simulink model "sixdof"  (R2019a)
settings: Solver=VariableStepAuto  StartTime=0.0  StopTime=15  RelTol=1e-3
InitFcn:
  | HeightAboveSeaLevel = 400 * rand;
  | Temperature = 288.15 + 30 * (rand - 0.5);
  | Pressure = 	101325 + 6000 * (rand - 0.5);
  | 
  | GustStart = 5 * rand;
  | GustLength = [100 + 50 * (rand - 0.5), 100 + 50 * (rand - 0.5), 100 + 50 * (rand - 0.5)];
  | GuestAmplitude = [ 10 * (rand - 0.5), 10 * (rand - 0.5),  10 * (rand - 0.5)];
  | 
  | ShearSpeed = 20 * rand;
  | ShearDirection = 360 * rand;
  | 
  | HeightAboveSeaLevel = 5.4419142084;
  | Temperature = 288.15;
  | Pressure = 	101325;
  | 
  | GustStart = 2.5;
  | GustLength = [100, 100, 100];
  | GuestAmplitude = [ 2.5, -2.5,  1];
  | 
  | ShearSpeed = 10;
  | ShearDirection = 180;
values from neighbouring files (symbols this model uses):
  cg = temp(4)    [NonlinearStateEstimationForActuatorDelay.m]
  D = zeros(size(B))    [RocketOutputFunction.m]    (also in StateSpaceController.m = zeros(13, 3); TimeDelayCompensationElevator.m = [0; 0])
  F = eye(6)    [MEKFAttitudeOnly.m]
  I = reshape(x(1:9), [3 3])    [AdaptiveLQR.m]    (also in MEKF.m = diag([0.08 0.08 0.002]); MEKFAttitudeOnly.m = diag([0.08 0.08 0.002]); MEKF_old.m = diag([0.08 0.08 0.002]); NonlinearStateEstimationForActuatorDelay.m = diag([Ixx, Ixx, Izz]))
  Ki2 = lqr(Ai2, Bi2, Q, R)    [StateSpaceController.m]
  mass = 1.0565    [ImpactVelocityNotParallelMatlab.m]    (also in NonlinearStateEstimationForActuatorDelay.m = temp(1); OneDLanding.m; RunImpactVelocityParforCompiled.m; Tracker.m = 1.0616753546)
  q = x(13:16)    [AdaptiveLQR.m]    (also in MEKF.m = nominal_state(4:7); MEKFAttitudeOnly.m = [1 0 0 0]; MEKF_old.m = nominal_state(4:7); NonlinearStateEstimationForActuatorDelay.m = x(4:7))
  r = sym('r', [3 1])    [StateSpaceController.m]    (also in TimeDelayCompensationElevator.m = [0;0]; Tracker.m = [0; 0; -(rocket_length - Average_cg)])
undefined symbols (not defined in the file or in its folder): Earth, Light, MIL, WGS84
libraries: aerolibutil x4, simulink x4, aerolibwind2 x3, aerolibfltsims x2, aerolibasang x2, shared6dof x1, aerolibatmos2 x1, aerolibbdyn x1, aerolibtransform2 x1, sharedtransform x1
settings Model: Creator=rahul  LastModifiedBy=rag
settings DataIOCC: ExternalInput=getinputstruct(op_trim34)  InitialState=getstatestruct(op_trim34)  ReturnWorkspaceOutputs=off
settings DebuggingCC: PregeneratedLibrarySubsystemCodeDiagnostic=none  ArithmeticOperatorsInVariantConditions=warning
settings SFSimCC: SimUseLocalCustomCode=off
settings RTWCC: RTWUseLocalCustomCode=off

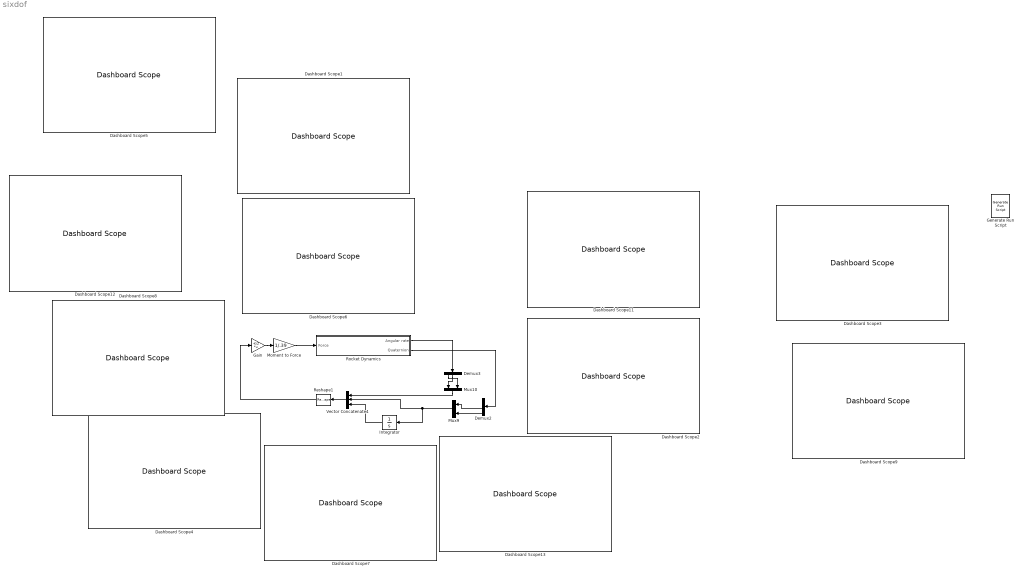
== system sixdof ==
  Dashboard Scope{1..9,11..13} (12 alike) : DashboardScope
  Demux2 : Demux
  Demux3 : Demux  Outputs=3
  Gain : Gain  Gain=-Ki2  Multiplication=Matrix(K*u)
  Generate Run Script : aerolibfltsims/Generate Run Script  Architecture=Win64  dataFlow=Send  GeometryModelName=c172p  AirportId=KSFO  RunwayId=10L  InitialAltitude=13  InitialHeading=113  OffsetDistance=4.72  OffsetAzimuth=0  InstallScenery=off  DisableShaders=off  OriginAddress=127.0.0.1  DestinationPort=5502  OriginPort=5505  LocalAddress=127.0.0.1  OutputFileName=runfg.bat  FlightGearBaseDirectory=C:\Program Files\FlightGear 2018.2.2
  Integrator : Integrator
  Moment to Force : Gain  Gain=1/.39
  Mux10 : Mux  Inputs=2
  Mux9 : Mux  Inputs=2
  Reshape1 : Reshape  OutputDimensionality=Column vector (2-D)
  Rocket Dynamics : Subsystem
  Vector Concatenate4 : Concatenate  NumInputs=3
  wires:
  Integrator/1 -> Vector Concatenate4/3
  Reshape1/1 -> Gain/1
  Demux2/3 -> Mux9/1
  Mux9/1 -> Integrator/1, Vector Concatenate4/2
  Vector Concatenate4/1 -> Reshape1/1
  Mux10/1 -> Vector Concatenate4/1
  Rocket Dynamics/1(Angular rate) -> Demux3/1
  Rocket Dynamics/2(Quaternion) -> Demux2/1
  Gain/1 -> Moment to Force/1
  Demux2/4 -> Mux9/2
  Demux3/2 -> Mux10/1
  Demux3/1 -> Mux10/2
  Moment to Force/1 -> Rocket Dynamics/1(Force)

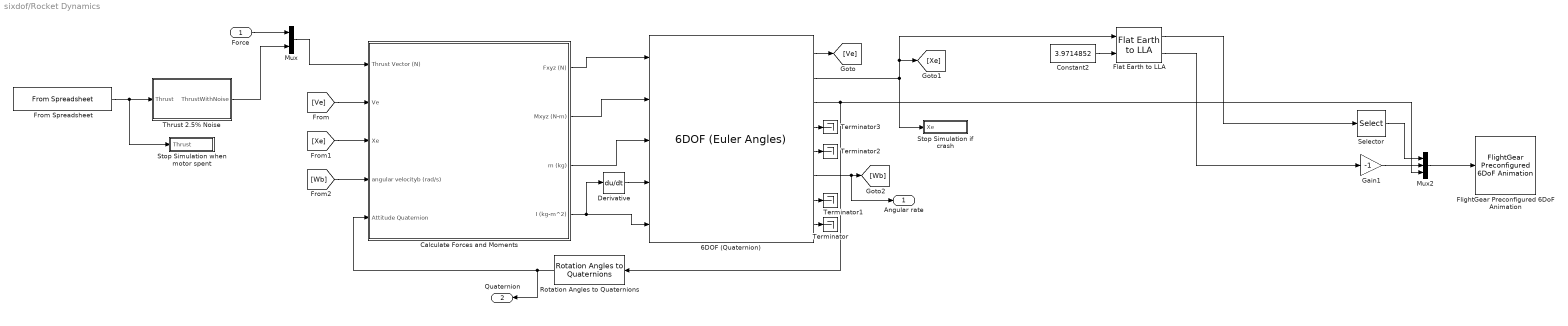
== system sixdof/Rocket Dynamics ==
  Force : Inport  PortDimensions=2
  6DOF (Quaternion) : shared6dof/6DOF (Euler Angles)  units=Metric (MKS)  mtype=Custom Variable  rep=Quaternion  xme_0=[0 0 0]  Vm_0=[0 0 0]  eul_0=[0 0 0]  pm_0=[0 0 0]  mass_0=1.0  mass_e=0.5  mass_f=2.0  inertia=eye(3)  inertia_e=eye(3)  inertia_f=2*eye(3)  k_quat=1.0  vre_flag=off  abi_flag=off  aMode=0  xme_statename=''  Vm_statename=''  eul_statename=''  quat_statename=''  pm_statename=''  mass_statename=''
      settings: SourceProductBaseCode=AE
  Calculate Forces and Moments : Subsystem
  Constant2 : Constant  Value=3.9714852
  Derivative : Derivative
  Flat Earth to LLA : aerolibtransform2/Flat Earth to LLA  units=Metric (MKS)  ptype=Earth (WGS84)  F=1/298.257223563  R=6378137  LL0=[21.318358277648 -157.9232805920725]  psi=052
  FlightGear Preconfigured 6DoF Animation : aerolibfltsims/FlightGear Preconfigured 6DoF Animation  xFlightGearVersion=v2018.2  DestinationIpAddress=127.0.0.1  DestinationPort=5502  SampleTime=1/30  packetVersion=24
      settings: SourceProductName=Aerospace Blockset
  From Spreadsheet : FromSpreadsheet  FileName=F10_Thrust.xls  ExtrapolationBeforeFirstDataPoint=Hold first value  ExtrapolationAfterLastDataPoint=Hold last value
  Gain1 : Gain  Gain=-1
  Mux : Mux  Inputs=2
  Mux2 : Mux  Inputs=3
  Rotation Angles to Quaternions : sharedtransform/Rotation Angles to Quaternions  rotationOrder=ZYX  aMode=aMode
      settings: SourceProductName=Aerospace Blockset  SourceProductBaseCode=AE
  Selector : Selector  InputPortWidth=2  IndexOptions=Index vector (dialog)  Indices=[2 1]  OutputSizes=1
  Stop Simulation if crash : Subsystem
  Stop Simulation when motor spent : Subsystem
  Terminator{,1..3} (4 alike) : Terminator
  Thrust 2.5% Noise : MATLAB Function  TreatAsAtomicUnit=on
  Angular rate : Outport
  Quaternion : Outport  Port=2
  wires:
  Derivative/1 -> 6DOF (Quaternion)/4
  6DOF (Quaternion)/6 -> Angular rate/1, [Wb]
  [Wb] -> Calculate Forces and Moments/4(angular velocityb (rad/s))
  Calculate Forces and Moments/3(m (kg)) -> 6DOF (Quaternion)/3
  6DOF (Quaternion)/4 -> Terminator3/1
  [Ve] -> Calculate Forces and Moments/2(Ve)
  6DOF (Quaternion)/7 -> Terminator1/1
  6DOF (Quaternion)/5 -> Terminator2/1
  Calculate Forces and Moments/1(Fxyz (N)) -> 6DOF (Quaternion)/1
  Calculate Forces and Moments/4(I (kg-m^2)) -> Derivative/1, 6DOF (Quaternion)/5
  [Xe] -> Calculate Forces and Moments/3(Xe)
  Rotation Angles to Quaternions/1 -> Quaternion/1, Calculate Forces and Moments/5(Attitude Quaternion)
  From Spreadsheet/1 -> Thrust 2.5% Noise/1(Thrust), Stop Simulation when motor spent/1(Thrust)
  6DOF (Quaternion)/1 -> [Ve]
  Calculate Forces and Moments/2(Mxyz (N-m)) -> 6DOF (Quaternion)/2
  6DOF (Quaternion)/8 -> Terminator/1
  Force/1 -> Mux/1
  Mux/1 -> Calculate Forces and Moments/1(Thrust Vector (N))
  Thrust 2.5% Noise/1(ThrustWithNoise) -> Mux/2
  Mux2/1 -> FlightGear Preconfigured 6DoF Animation/1
  Constant2/1 -> Flat Earth to LLA/2
  Flat Earth to LLA/2 -> Gain1/1
  Flat Earth to LLA/1 -> Selector/1
  Gain1/1 -> Mux2/2
  6DOF (Quaternion)/3 -> Mux2/3, Rotation Angles to Quaternions/1
  Selector/1 -> Mux2/1
  6DOF (Quaternion)/2 -> Stop Simulation if crash/1(Xe), [Xe], Flat Earth to LLA/1

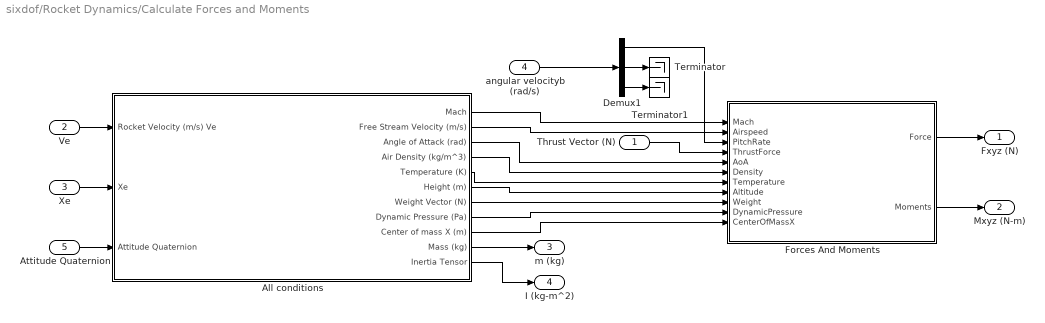
== system sixdof/Rocket Dynamics/Calculate Forces and Moments ==
  Thrust Vector (N) : Inport
  Ve : Inport  Port=2
  Xe : Inport  Port=3
  angular velocityb (rad/s) : Inport  Port=4
  Attitude Quaternion : Inport  Port=5
  All conditions : Subsystem
  Demux1 : Demux  Outputs=3
  Forces And Moments : MATLAB Function  TreatAsAtomicUnit=on
  Terminator : Terminator
  Terminator1 : Terminator
  Fxyz (N) : Outport
  Mxyz (N-m) : Outport  Port=2
  m (kg) : Outport  Port=3
  I (kg-m^2) : Outport  Port=4
  wires:
  Demux1/1 -> Forces And Moments/3(PitchRate)
  All conditions/11(Inertia Tensor) -> I (kg-m^2)/1
  All conditions/2(Free Stream Velocity (m/s)) -> Forces And Moments/2(Airspeed)
  All conditions/9(Center of mass X (m)) -> Forces And Moments/11(CenterOfMassX)
  All conditions/5(Temperature (K)) -> Forces And Moments/7(Temperature)
  Xe/1 -> All conditions/2(Xe)
  angular velocityb (rad/s)/1 -> Demux1/1
  All conditions/3(Angle of Attack (rad)) -> Forces And Moments/5(AoA)
  All conditions/1(Mach) -> Forces And Moments/1(Mach)
  All conditions/4(Air Density (kg/m^3)) -> Forces And Moments/6(Density)
  All conditions/8(Dynamic Pressure (Pa)) -> Forces And Moments/10(DynamicPressure)
  All conditions/6(Height (m)) -> Forces And Moments/8(Altitude)
  All conditions/7(Weight Vector (N)) -> Forces And Moments/9(Weight)
  Thrust Vector (N)/1 -> Forces And Moments/4(ThrustForce)
  Attitude Quaternion/1 -> All conditions/3(Attitude Quaternion)
  Ve/1 -> All conditions/1(Rocket Velocity (m/s) Ve)
  All conditions/10(Mass (kg)) -> m (kg)/1
  Demux1/2 -> Terminator/1
  Demux1/3 -> Terminator1/1
  Forces And Moments/1(Force) -> Fxyz (N)/1
  Forces And Moments/2(Moments) -> Mxyz (N-m)/1

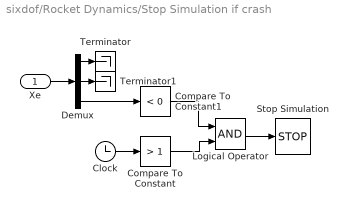
== system sixdof/Rocket Dynamics/Stop Simulation if crash ==
  Xe : Inport
  Clock : Clock
  Compare To Constant : simulink/Logic and Bit Operations/Compare To Constant  relop=>  const=1  OutDataTypeStr=boolean
  Compare To Constant1 : simulink/Logic and Bit Operations/Compare To Constant  relop=<  const=0  OutDataTypeStr=boolean
  Demux : Demux  Outputs=3
  Logical Operator : Logic  AllPortsSameDT=off  OutDataTypeStr=boolean
  Stop Simulation : Stop
  Terminator : Terminator
  Terminator1 : Terminator
  wires:
  Logical Operator/1 -> Stop Simulation/1
  Compare To Constant/1 -> Logical Operator/2
  Clock/1 -> Compare To Constant/1
  Compare To Constant1/1 -> Logical Operator/1
  Xe/1 -> Demux/1
  Demux/1 -> Terminator/1
  Demux/2 -> Terminator1/1
  Demux/3 -> Compare To Constant1/1

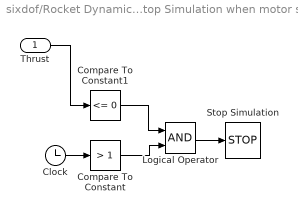
== system sixdof/Rocket Dynamics/Stop Simulation when motor spent ==
  Thrust : Inport
  Clock : Clock
  Compare To Constant : simulink/Logic and Bit Operations/Compare To Constant  relop=>  const=1  OutDataTypeStr=boolean
  Compare To Constant1 : simulink/Logic and Bit Operations/Compare To Constant  relop=<=  const=0  OutDataTypeStr=boolean
  Logical Operator : Logic  AllPortsSameDT=off  OutDataTypeStr=boolean
  Stop Simulation : Stop
  wires:
  Logical Operator/1 -> Stop Simulation/1
  Compare To Constant/1 -> Logical Operator/2
  Clock/1 -> Compare To Constant/1
  Compare To Constant1/1 -> Logical Operator/1
  Thrust/1 -> Compare To Constant1/1

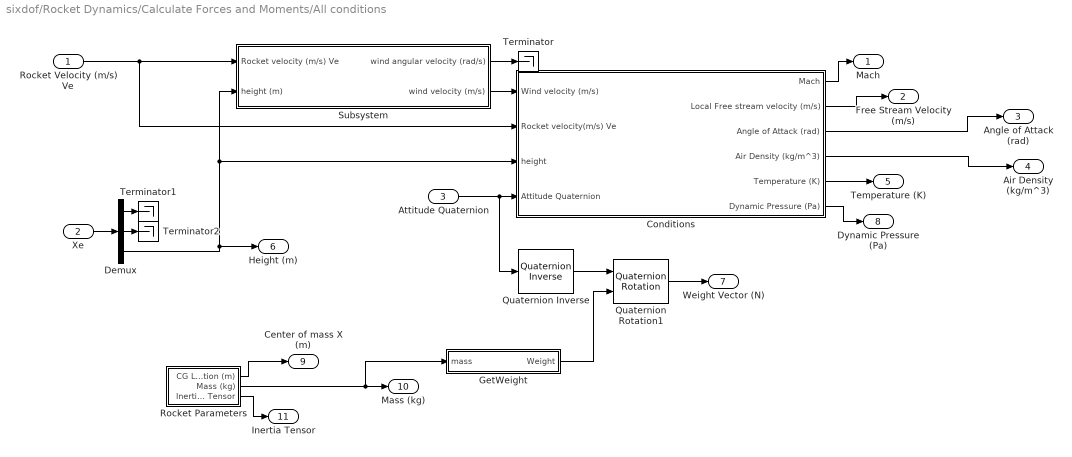
== system sixdof/Rocket Dynamics/Calculate Forces and Moments/All conditions ==
  Rocket Velocity (m/s) Ve : Inport
  Xe : Inport  Port=2
  Attitude Quaternion : Inport  Port=3
  Conditions : Subsystem
  Demux : Demux  Outputs=3
  GetWeight : MATLAB Function  TreatAsAtomicUnit=on
  Quaternion Inverse : aerolibutil/Quaternion Inverse
      settings: SourceProductName=Aerospace Blockset
  Quaternion Rotation1 : aerolibutil/Quaternion Rotation
  Rocket Parameters : Subsystem
  Subsystem : Subsystem
  Terminator : Terminator
  Terminator1 : Terminator
  Terminator2 : Terminator
  Mach : Outport
  Free Stream Velocity (m/s) : Outport  Port=2
  Angle of Attack (rad) : Outport  Port=3
  Air Density (kg/m^3) : Outport  Port=4
  Temperature (K) : Outport  Port=5
  Height (m) : Outport  Port=6
  Weight Vector (N) : Outport  Port=7
  Dynamic Pressure (Pa) : Outport  Port=8
  Center of mass X (m) : Outport  Port=9
  Mass (kg) : Outport  Port=10
  Inertia Tensor : Outport  Port=11
  wires:
  Demux/3 -> Subsystem/2(height (m)), Conditions/3(height), Height (m)/1
  Conditions/4(Air Density (kg/m^3)) -> Air Density (kg/m^3)/1
  Rocket Velocity (m/s) Ve/1 -> Conditions/2(Rocket velocity(m/s) Ve), Subsystem/1(Rocket velocity (m/s) Ve)
  Conditions/5(Temperature (K)) -> Temperature (K)/1
  Conditions/1(Mach) -> Mach/1
  Subsystem/1(wind angular velocity (rad/s)) -> Terminator/1
  Conditions/2(Local Free stream velocity (m/s)) -> Free Stream Velocity (m/s)/1
  Demux/2 -> Terminator2/1
  GetWeight/1(Weight) -> Quaternion Rotation1/2
  Xe/1 -> Demux/1
  Rocket Parameters/1(CG Location (m)) -> Center of mass X (m)/1
  Rocket Parameters/3(Inertia Tensor) -> Inertia Tensor/1
  Quaternion Rotation1/1 -> Weight Vector (N)/1
  Conditions/3(Angle of Attack (rad)) -> Angle of Attack (rad)/1
  Demux/1 -> Terminator1/1
  Conditions/6(Dynamic Pressure (Pa)) -> Dynamic Pressure (Pa)/1
  Rocket Parameters/2(Mass (kg)) -> GetWeight/1(mass), Mass (kg)/1
  Subsystem/2(wind velocity (m/s)) -> Conditions/1(Wind velocity (m/s))
  Quaternion Inverse/1 -> Quaternion Rotation1/1
  Attitude Quaternion/1 -> Quaternion Inverse/1, Conditions/4(Attitude Quaternion)

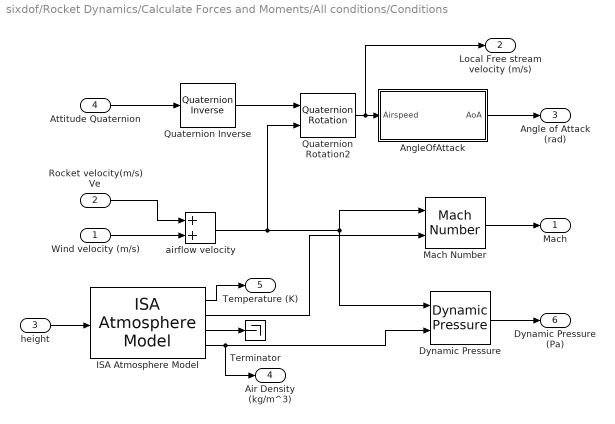
== system sixdof/Rocket Dynamics/Calculate Forces and Moments/All conditions/Conditions ==
  Wind velocity (m/s) : Inport
  Rocket velocity(m/s) Ve : Inport  Port=2
  height : Inport  Port=3
  Attitude Quaternion : Inport  Port=4
  AngleOfAttack : MATLAB Function  TreatAsAtomicUnit=on
  Dynamic Pressure : aerolibasang/Dynamic Pressure
  ISA Atmosphere Model : aerolibatmos2/ISA Atmosphere Model  custom=on  g=9.80665  gamma=1.4  R=287.0531  L=0.0065  h_trop=11000  h_strat=20000  rho0=1.225  P0=Pressure  T0=Temperature  h0=0
      settings: SourceProductName=Aerospace Blockset
  Mach Number : aerolibasang/Mach Number
      settings: SourceProductName=Aerospace Blockset  SourceProductBaseCode=AE
  Quaternion Inverse : aerolibutil/Quaternion Inverse
      settings: SourceProductName=Aerospace Blockset
  Quaternion Rotation2 : aerolibutil/Quaternion Rotation
  Terminator : Terminator
  airflow velocity : Sum
  Mach : Outport
  Local Free stream velocity (m/s) : Outport  Port=2
  Angle of Attack (rad) : Outport  Port=3
  Air Density (kg/m^3) : Outport  Port=4
  Temperature (K) : Outport  Port=5
  Dynamic Pressure (Pa) : Outport  Port=6
  wires:
  airflow velocity/1 -> Quaternion Rotation2/2, Dynamic Pressure/1, Mach Number/1
  Quaternion Rotation2/1 -> AngleOfAttack/1(Airspeed), Local Free stream velocity (m/s)/1
  ISA Atmosphere Model/4 -> Dynamic Pressure/2, Air Density (kg/m^3)/1
  ISA Atmosphere Model/2 -> Mach Number/2
  Dynamic Pressure/1 -> Dynamic Pressure (Pa)/1
  ISA Atmosphere Model/3 -> Terminator/1
  Mach Number/1 -> Mach/1
  Rocket velocity(m/s) Ve/1 -> airflow velocity/1
  ISA Atmosphere Model/1 -> Temperature (K)/1
  AngleOfAttack/1(AoA) -> Angle of Attack (rad)/1
  height/1 -> ISA Atmosphere Model/1
  Attitude Quaternion/1 -> Quaternion Inverse/1
  Wind velocity (m/s)/1 -> airflow velocity/2
  Quaternion Inverse/1 -> Quaternion Rotation2/1

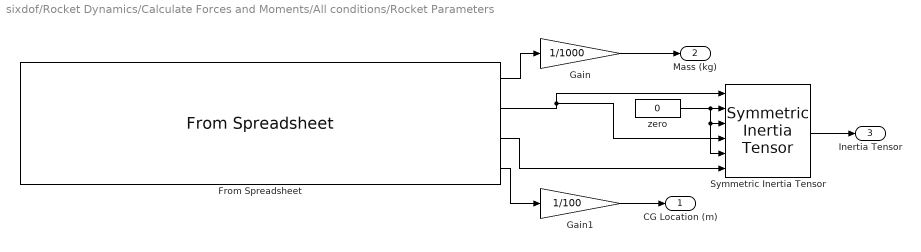
== system sixdof/Rocket Dynamics/Calculate Forces and Moments/All conditions/Rocket Parameters ==
  From Spreadsheet : FromSpreadsheet  FileName=mass,cg,I.xlsx  SheetName=mass,cg,I  Range=A1:E251  ExtrapolationBeforeFirstDataPoint=Hold first value  ExtrapolationAfterLastDataPoint=Hold last value
  Gain : Gain  Gain=1/1000
  Gain1 : Gain  Gain=1/100
  Symmetric Inertia Tensor : aerolibbdyn/Symmetric Inertia Tensor
      settings: SourceProductName=Aerospace Blockset  SourceProductBaseCode=AE
  zero : Constant  Value=0
  CG Location (m) : Outport
  Mass (kg) : Outport  Port=2
  Inertia Tensor : Outport  Port=3
  wires:
  zero/1 -> Symmetric Inertia Tensor/5, Symmetric Inertia Tensor/3, Symmetric Inertia Tensor/2
  From Spreadsheet/2 -> Symmetric Inertia Tensor/1, Symmetric Inertia Tensor/4
  From Spreadsheet/3 -> Symmetric Inertia Tensor/6
  Symmetric Inertia Tensor/1 -> Inertia Tensor/1
  From Spreadsheet/4 -> Gain1/1
  From Spreadsheet/1 -> Gain/1
  Gain/1 -> Mass (kg)/1
  Gain1/1 -> CG Location (m)/1

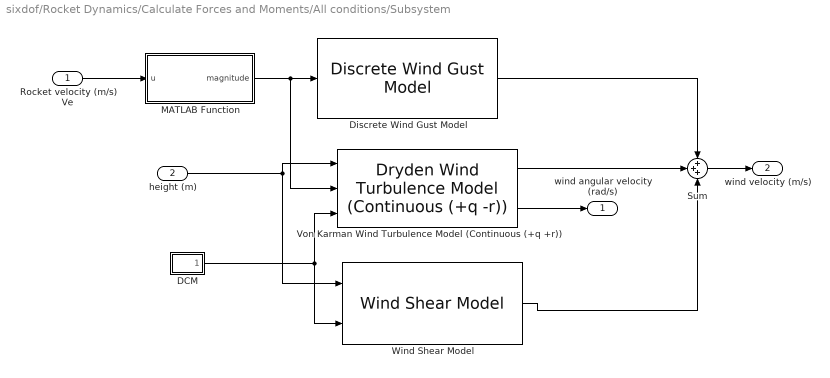
== system sixdof/Rocket Dynamics/Calculate Forces and Moments/All conditions/Subsystem ==
  Rocket velocity (m/s) Ve : Inport
  height (m) : Inport  Port=2
  DCM : MATLAB Function  TreatAsAtomicUnit=on
  Discrete Wind Gust Model : aerolibwind2/Discrete Wind Gust Model  units=Metric (MKS)  Gx=on  Gy=on  Gz=on  t_0=GustStart  d_m=GustLength  v_m=GuestAmplitude
      settings: SourceProductName=Aerospace Blockset
  MATLAB Function : MATLAB Function  TreatAsAtomicUnit=on
  Sum : Sum  Inputs=3
  Von Karman Wind Turbulence Model (Continuous (+q +r)) : aerolibwind2/Dryden Wind Turbulence Model  (Continuous (+q -r))  units=Metric (MKS)  spec=MIL-F-8785C  model=Discrete Dryden (+q -r)  W20=ShearSpeed  Wdeg=ShearDirection  TurbProb=10^-2 - Light  L_high=762  Wingspan=10  ts=0.1  Seed=[23341 23342 23343 23344]  T_on=on
      settings: SourceProductName=Aerospace Blockset
  Wind Shear Model : aerolibwind2/Wind Shear Model  units=Metric (MKS)  phase=Category C - Terminal Flight Phase  W_20=ShearSpeed  Wdeg=ShearDirection
      settings: SourceProductName=Aerospace Blockset
  wind angular velocity (rad/s) : Outport
  wind velocity (m/s) : Outport  Port=2
  wires:
  height (m)/1 -> Wind Shear Model/1, Von Karman Wind Turbulence Model (Continuous (+q +r))/1
  Discrete Wind Gust Model/1 -> Sum/1
  DCM/1(DCM) -> Von Karman Wind Turbulence Model (Continuous (+q +r))/3, Wind Shear Model/2
  MATLAB Function/1(magnitude) -> Von Karman Wind Turbulence Model (Continuous (+q +r))/2, Discrete Wind Gust Model/1
  Sum/1 -> wind velocity (m/s)/1
  Wind Shear Model/1 -> Sum/3
  Von Karman Wind Turbulence Model (Continuous (+q +r))/1 -> Sum/2
  Von Karman Wind Turbulence Model (Continuous (+q +r))/2 -> wind angular velocity (rad/s)/1
  Rocket velocity (m/s) Ve/1 -> MATLAB Function/1(u)

== matlab function sixdof/Rocket Dynamics/Calculate Forces and Moments/All conditions/Conditions/AngleOfAttack ==
  settings: updateMethod=DISCRETE
  data: Airspeed input; AoA output
function AoA = AngleOfAttack(Airspeed)
    AoA = acos(Airspeed(3) / norm(Airspeed)); 
    
    if norm(Airspeed) <= .01
        AoA = 0;
    end
end

== matlab function sixdof/Rocket Dynamics/Calculate Forces and Moments/All conditions/GetWeight ==
  settings: updateMethod=DISCRETE
  data: Weight output; mass input
function Weight  = MassToWeight(mass)
   Weight = [0; 0; -9.8065*mass];
   end

== matlab function sixdof/Rocket Dynamics/Calculate Forces and Moments/All conditions/Subsystem/DCM ==
  settings: updateMethod=DISCRETE
  data: DCM output
function DCM  = forces
    DCM = [1,0,0;0,1,0;0,0,1];

== matlab function sixdof/Rocket Dynamics/Calculate Forces and Moments/All conditions/Subsystem/MATLAB Function ==
  data: u input; magnitude output
function magnitude = VectorNorm(u)
    magnitude = norm(u);

== matlab function sixdof/Rocket Dynamics/Calculate Forces and Moments/Forces And Moments ==
  settings: updateMethod=DISCRETE
  data: Mach input; Airspeed input; PitchRate input; ThrustForce input; AoA input; Density input; Temperature input; Altitude input; Weight input; Force output; DynamicPressure input; Moments output; CenterOfMassX input
function [Force, Moments] = forces(Mach, Airspeed, PitchRate, ThrustForce, AoA, Density, Temperature, Altitude, Weight, DynamicPressure, CenterOfMassX)
    %% Rocket Shape Constants
    Reference_Diameter = 7.62e-2;
    Reference_Radius = Reference_Diameter / 2;
    Reference_Area = Reference_Radius^2 * pi;
    
    NoseCone_Length = 15e-2;
    BodyTube_Length = 80e-2;
    NoseCone_WetArea = pi * Reference_Radius * NoseCone_Length;          % pi*r*l
    BodyTube_WetArea = pi * Reference_Radius * 2 * BodyTube_Length;      % pi*d*l
    NoseCone_PlanformArea = Reference_Diameter * NoseCone_Length / 2;
    BodyTube_PlanformArea = Reference_Diameter * BodyTube_Length;
    
    SurfaceRoughness = 20e-6;
    
    sinphi = Reference_Radius / hypot(Reference_Radius, NoseCone_Length);
    BodyTube_CP = 0.55;
    NoseCone_CP = 0.1;
    PitchCenterX = 0;
    
    % Random Noise
    SurfaceRoughness = SurfaceRoughness + 20e-6 * (rand - 0.5); % =- 10 um
    CenterOfMassX = CenterOfMassX + .04 * (rand - 0.5); % +- 2cm 
    
    COT_to_COM = .95 - CenterOfMassX; %get actual value and change over time as solid motor burns
    COT_to_COM = COT_to_COM + .02 * (rand - 0.5); 
    
    %% General Constants
    K = 1.1;
   
    %% Coefficients
    [CN, Cpitch] = CalculatePitchAndNormalCDs(K, Reference_Diameter, AoA, Airspeed, PitchRate, NoseCone_Length, BodyTube_Length, Reference_Area, CenterOfMassX, PitchCenterX, NoseCone_PlanformArea, BodyTube_PlanformArea, NoseCone_CP, BodyTube_CP);
    
    Cbase = .12 + .13*Mach^2;
    CFrictionDrag = CalculateFrictionDrag(Temperature, Density, Reference_Radius, Reference_Area, SurfaceRoughness, NoseCone_Length, BodyTube_Length, Airspeed, Mach, NoseCone_WetArea, BodyTube_WetArea);
    Cpressure = PressureDragForce(sinphi);
    
    Cdrag = Cbase + CFrictionDrag + Cpressure;
    Caxial = AxialDragMul(AoA) * Cdrag;
    
    Cyaw = 0.0;
    
    Croll = 0;
    Cside = 0;
    
    %% Random Noise to pitch and yaw coefficients in the range of +- 5e-4
    Cpitch = Cpitch + .1 * (rand - 0.5);
    Cyaw = Cyaw + .1 * (rand - 0.5);
    Croll = Croll + .1 * (rand - 0.5);
    
    %% Forces and Moments
    z = DynamicPressure * Reference_Area;
        
    lengtha = norm(Airspeed(1:2));
    trig = Airspeed(1:2) / lengtha;

    ThetaRotation = [trig(1), -trig(2), 0; trig(2), trig(1), 0; 0 0 1];
    
    Force = -z * ThetaRotation * [CN; Cside; Caxial] + ThrustForce + Weight;
    
    if Altitude <= 0 && Force(3) < 0
        Force(3) = 0;
    end
    
    Thrust_moment = COT_to_COM * [ThrustForce(2); ThrustForce(1); 0];
    Moments = z * Reference_Diameter * ThetaRotation * [-Cyaw; Cpitch; Croll] + Thrust_moment;
end

== matlab function sixdof/Rocket Dynamics/Thrust 2.5% Noise ==
  settings: updateMethod=DISCRETE
  data: ThrustWithNoise output; Thrust input
function ThrustWithNoise  = AddNoiseToThrust(Thrust)
   ThrustWithNoise = (Thrust + Thrust * 0.025 * (rand - 0.5));
   end
